simulink model "LAB9_PI"  (R2022b)
settings: Solver=VariableStepAuto  StartTime=0.0  StopTime=czas_systemu  RelTol=1e-3
values from neighbouring files (symbols this model uses):
  Cvp = cp*rop*Vp    (= 36000)    [LAB9.m]
  Cvw = cp*rop*Vw    (= 72000)    [LAB9.m]
  dqg = 0.1*q_g_N    (= 1000)    [LAB9.m]
  dTzew = 1    [LAB9.m]
  K_cp = ((a1*q_g_N)*(T_wew_N-Tp_N))/((Tp_N-T_zew_N)*(T_wew_N-T_zew_N+a1*(T_wew_N-Tp_N)))    (= 23.2558139535)    [LAB9.m]
  K_cw = (q_g_N)/(T_wew_N-T_zew_N+a1*(T_wew_N-Tp_N))    (= 232.558139535)    [LAB9.m]
  K_cwp = (a1*(q_g_N))/(T_wew_N-T_zew_N+a1*(T_wew_N-Tp_N))    (= 69.7674418605)    [LAB9.m]
  Kd = 0    [LAB9.m]
  Ki = Kp/(3.33*T_0_tp)    (= 9.00900900901)    [LAB9.m]
  Kp = (0.9*T_sp)/(ksTp*T_0_tp)    (= 3000)    [LAB9.m]
  L11 = [ksTwew]    [LAB9.m]
  L12 = [ksTp]    [LAB9.m]
  L21 = [kmdTwew]    [LAB9.m]
  L22 = [kmdTp]    [LAB9.m]
  M1 = [T,1]    [LAB9.m]
  M2 = [T_sp,1]    [LAB9.m]
  M3 = [T2,1]    [LAB9.m]
  M4 = [T3,1]    [LAB9.m]
  q_g_0 = K_cw*(T_wew_0-T_zew_0)+K_cwp*(T_wew_0-Tp_0)    (= 11666.6666667)    [LAB9.m]
  t0 = 1000    [LAB9.m]
  T_0_tp = 100    [LAB9.m]
  T_0_wew = 0    [LAB9.m]
  T_wew_0 = (K_cwp*Tp_0+K_cp*Tp_0-K_cp*T_zew_0)/K_cwp    (= 26.6666666667)    [LAB9.m]
  T_zew_0 = T_zew_N    (= -20)    [LAB9.m]
  To = t_2w-T2    (= 0)    [LAB9.m]
  To1 = t_2p-T3    (= 175)    [LAB9.m]
  Tp_0 = Tp_N+b    (= 15)    [LAB9.m]
  Tp_N = 10    [LAB9.m]
libraries: slpidlib x5
settings Model: Creator=maciejrudy  LastModifiedBy=Dawid
settings SolverCC: AlgebraicLoopSolver=TrustRegion
settings DataIOCC: ReturnWorkspaceOutputs=off
settings DebuggingCC: UnconnectedInputMsg=warning  UnconnectedOutputMsg=warning  UnconnectedLineMsg=warning  SFMachineParentedDataDiag=warning
settings ModelReferenceCC: EnableRefExpFcnMdlSchedulingChecks=on
settings RTWCC: DLArmComputeVersion=19.05

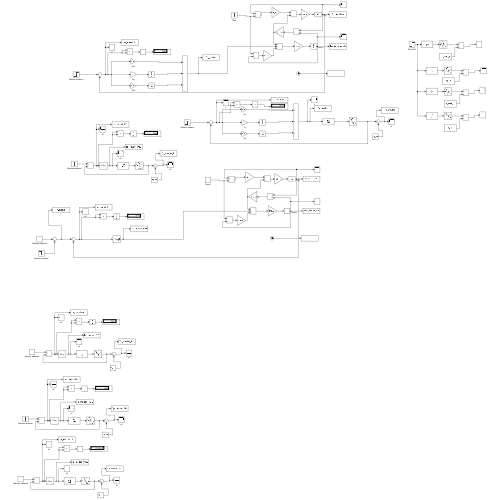
[thumbnail: Simulink's stored preview of the top-level diagram]
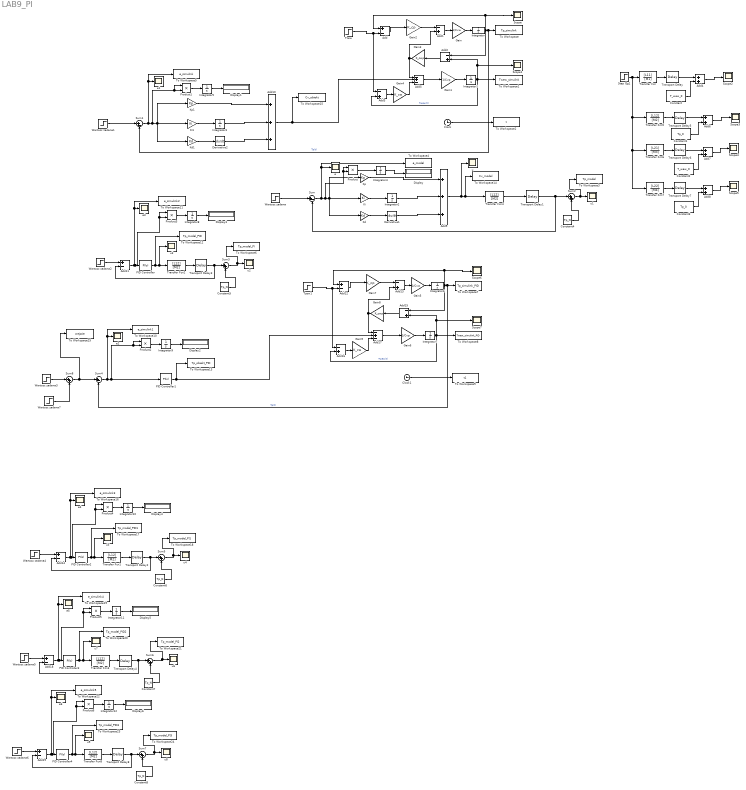
== system LAB9_PI ==
  Add{,11..12,14,18..19} (6 alike) : Sum  Inputs=+-
  Add{1..3,13,15..16} (6 alike) : Sum  Inputs=-+
  Add10 : Sum  Inputs=+++
  Add17 : Sum  Inputs=-+-
  Add{4,6..8} (4 alike) : Sum
  Add5 : Sum  Inputs=-+-
  Add9 : Sum  Inputs=+++
  Clock : Clock
  Clock1 : Clock
  Constant : Constant  Value=T_wew_0
  Constant1 : Constant  Value=Tp_0
  Constant2 : Constant  Value=T_wew_0
  Constant3 : Constant  Value=Tp_0
  Constant{4..8} (5 alike) : Constant  Value=Tp_N
  Derivative1 : Derivative
  Derivative2 : Derivative
  Display{,1..6} (7 alike) : Display
  Gain : Gain  Gain=1/Cvw
  Gain1 : Gain  Gain=1/Cvp
  Gain2 : Gain  Gain=K_cp
  Gain3 : Gain  Gain=K_cwp
  Gain4 : Gain  Gain=K_cw
  Gain5 : Gain  Gain=1/Cvw
  Gain6 : Gain  Gain=1/Cvp
  Gain7 : Gain  Gain=K_cp
  Gain8 : Gain  Gain=K_cwp
  Gain9 : Gain  Gain=K_cw
  Integrator : Integrator  InitialCondition=Tp_0
  Integrator1 : Integrator  InitialCondition=T_wew_0
  Integrator{2,4..5,8..12} (8 alike) : Integrator
  Integrator3 : Integrator  InitialCondition=q_g_0
  Integrator6 : Integrator  InitialCondition=Tp_0
  Integrator7 : Integrator  InitialCondition=T_wew_0
  Kd : Gain  Gain=Kd
  Kd1 : Gain  Gain=Kd
  Ki : Gain  Gain=Ki
  Ki1 : Gain  Gain=Ki
  Kp : Gain  Gain=Kp
  Kp1 : Gain  Gain=Kp
  PID Controller : slpidlib/PID Controller  Controller=PI  Form=Parallel  TimeDomain=Continuous-time  UseExternalTs=off  SampleTime=-1  IntegratorMethod=Forward Euler  FilterMethod=Forward Euler  ControllerParametersSource=internal  P=474.217741938703  I=1.00741516642566  UseKiTs=off  D=-0.04857589160968  N=3.78094165182863  UseFilter=on  TunerSelectOption=Transfer Function Based (PID Tuner App)  InitialConditionSource=internal  InitialConditionForIntegrator=0  InitialConditionForFilter=0  DifferentiatorICPrevScaledInput=0  ExternalReset=none  TrackingMode=off  Kt=1  LimitOutput=off  SatLimitsSource=internal  UpperSaturationLimit=inf  LowerSaturationLimit=-inf  LinearizeAsGain=on  AntiWindupMode=none  Kb=1  LimitIntegrator=off  UpperIntegratorSaturationLimit=inf  LowerIntegratorSaturationLimit=-inf  POutMin=[]  POutMax=[]  IOutMin=[]  IOutMax=[]  DOutMin=[]  DOutMax=[]  NOutMin=[]  NOutMax=[]  SumOutMin=[]  SumOutMax=[]  SaturationOutMin=[]  SaturationOutMax=[]  PParamMin=[]  PParamMax=[]  IParamMin=[]  IParamMax=[]  DParamMin=[]  DParamMax=[]  NParamMin=[]  NParamMax=[]  KbParamMin=[]  KbParamMax=[]  KtParamMin=[]  KtParamMax=[]  KbOutMin=[]  KbOutMax=[]  KtOutMin=[]  KtOutMax=[]  IntegratorOutMin=[]  IntegratorOutMax=[]  FilterOutMin=[]  FilterOutMax=[]  SumI1OutMin=[]  SumI1OutMax=[]  SumI2OutMin=[]  SumI2OutMax=[]  SumI3OutMin=[]  SumI3OutMax=[]  SumI4OutMin=[]  SumI4OutMax=[]  SumDOutMin=[]  SumDOutMax=[]  DifferentiatorOutMin=[]  DifferentiatorOutMax=[]  FilterDiffOutCoefMin=[]  FilterDiffOutCoefMax=[]  ReciprocalOutMin=[]  ReciprocalOutMax=[]  SumDenOutMin=[]  SumDenOutMax=[]  SumNumOutMin=[]  SumNumOutMax=[]  DivideOutMin=[]  DivideOutMax=[]  UdiffTsProdOutMin=[]  UdiffTsProdOutMax=[]  NTsProdOutMin=[]  NTsProdOutMax=[]  UintegralTsProdOutMin=[]  UintegralTsProdOutMax=[]  UngainTsProdOutMin=[]  UngainTsProdOutMax=[]  ClampingZeroOutDataTypeStr=Inherit: Inherit via back propagation  ClampingZeroOutMin=[]  ClampingZeroOutMax=[]  FilterDenConstantOutDataTypeStr=Inherit: Inherit via back propagation  FilterDenConstantOutMin=[]  FilterDenConstantOutMax=[]  PCopyOutDataTypeStr=Inherit: Inherit via back propagation  PCopyOutMin=[]  PCopyOutMax=[]  NCopyOutDataTypeStr=Inherit: Inherit via back propagation  NCopyOutMin=[]  NCopyOutMax=[]  IntegratorContinuousStateAttributes=''  IntegratorStateMustResolveToSignalObject=off  IntegratorRTWStateStorageClass=Auto  FilterContinuousStateAttributes=''  FilterStateMustResolveToSignalObject=off  FilterRTWStateStorageClass=Auto  ParallelPVariant=InternalParameters  IdealPVariant=Disabled  IVariant=InternalParameters  DVariant=Disabled  IntegratorVariant=Continuous  SatVariant=Disabled  AWVariant=Passthrough  PCopyVariant=Disabled  TRVariant=Disabled  FdbkBlocksVariant=Forward  IdealPFdbkVariant=Disabled  SatFdbkVariant=Disabled  DerivativeFilterVariant=Disabled  NVariant=Disabled  NCopyVariant=Disabled_SignalSpec  FilterICVariant=Disabled  IntegratorICVariant=InternalICs  ExternalResetVariant=Disabled  TRSumVariant=Passthrough  SumFdbkVariant=Disabled  SumVariant=Sum_PI  TsampFilterVariant=InternalTs  TsampNgainVariant=Passthrough  TsampIntegralVariant=Passthrough  ExternalSaturationOutDataTypeStr=Inherit: Same as second input
  PID Controller1 : slpidlib/PID Controller  Controller=PI  Form=Parallel  TimeDomain=Continuous-time  UseExternalTs=off  SampleTime=-1  IntegratorMethod=Forward Euler  FilterMethod=Forward Euler  ControllerParametersSource=internal  P=2025.02642427682  I=9.10127320670196  UseKiTs=off  D=-0.04857589160968  N=3.78094165182863  UseFilter=on  TunerSelectOption=Transfer Function Based (PID Tuner App)  InitialConditionSource=internal  InitialConditionForIntegrator=q_g_0  InitialConditionForFilter=0  DifferentiatorICPrevScaledInput=0  ExternalReset=none  TrackingMode=off  Kt=1  LimitOutput=on  SatLimitsSource=internal  UpperSaturationLimit=13000  LowerSaturationLimit=-inf  LinearizeAsGain=on  AntiWindupMode=back-calculation  Kb=2  LimitIntegrator=off  UpperIntegratorSaturationLimit=inf  LowerIntegratorSaturationLimit=-inf  POutMin=[]  POutMax=[]  IOutMin=[]  IOutMax=[]  DOutMin=[]  DOutMax=[]  NOutMin=[]  NOutMax=[]  SumOutMin=[]  SumOutMax=[]  SaturationOutMin=[]  SaturationOutMax=[]  PParamMin=[]  PParamMax=[]  IParamMin=[]  IParamMax=[]  DParamMin=[]  DParamMax=[]  NParamMin=[]  NParamMax=[]  KbParamMin=[]  KbParamMax=[]  KtParamMin=[]  KtParamMax=[]  KbOutMin=[]  KbOutMax=[]  KtOutMin=[]  KtOutMax=[]  IntegratorOutMin=[]  IntegratorOutMax=[]  FilterOutMin=[]  FilterOutMax=[]  SumI1OutMin=[]  SumI1OutMax=[]  SumI2OutMin=[]  SumI2OutMax=[]  SumI3OutMin=[]  SumI3OutMax=[]  SumI4OutMin=[]  SumI4OutMax=[]  SumDOutMin=[]  SumDOutMax=[]  DifferentiatorOutMin=[]  DifferentiatorOutMax=[]  FilterDiffOutCoefMin=[]  FilterDiffOutCoefMax=[]  ReciprocalOutMin=[]  ReciprocalOutMax=[]  SumDenOutMin=[]  SumDenOutMax=[]  SumNumOutMin=[]  SumNumOutMax=[]  DivideOutMin=[]  DivideOutMax=[]  UdiffTsProdOutMin=[]  UdiffTsProdOutMax=[]  NTsProdOutMin=[]  NTsProdOutMax=[]  UintegralTsProdOutMin=[]  UintegralTsProdOutMax=[]  UngainTsProdOutMin=[]  UngainTsProdOutMax=[]  ClampingZeroOutDataTypeStr=Inherit: Inherit via back propagation  ClampingZeroOutMin=[]  ClampingZeroOutMax=[]  FilterDenConstantOutDataTypeStr=Inherit: Inherit via back propagation  FilterDenConstantOutMin=[]  FilterDenConstantOutMax=[]  PCopyOutDataTypeStr=Inherit: Inherit via back propagation  PCopyOutMin=[]  PCopyOutMax=[]  NCopyOutDataTypeStr=Inherit: Inherit via back propagation  NCopyOutMin=[]  NCopyOutMax=[]  IntegratorContinuousStateAttributes=''  IntegratorStateMustResolveToSignalObject=off  IntegratorRTWStateStorageClass=Auto  FilterContinuousStateAttributes=''  FilterStateMustResolveToSignalObject=off  FilterRTWStateStorageClass=Auto  ParallelPVariant=InternalParameters  IdealPVariant=Disabled  IVariant=InternalParameters  DVariant=Disabled  IntegratorVariant=Continuous  SatVariant=Enabled  AWVariant=BackCalculation  PCopyVariant=Disabled  TRVariant=Disabled  FdbkBlocksVariant=Forward  IdealPFdbkVariant=Disabled  SatFdbkVariant=Disabled  DerivativeFilterVariant=Disabled  NVariant=Disabled  NCopyVariant=Disabled_SignalSpec  FilterICVariant=Disabled  IntegratorICVariant=InternalICs  ExternalResetVariant=Disabled  TRSumVariant=Passthrough  SumFdbkVariant=Disabled  SumVariant=Sum_PI  TsampFilterVariant=InternalTs  TsampNgainVariant=Passthrough  TsampIntegralVariant=Passthrough  ExternalSaturationOutDataTypeStr=Inherit: Same as second input
  PID Controller2 : slpidlib/PID Controller  Controller=PI  Form=Parallel  TimeDomain=Continuous-time  UseExternalTs=off  SampleTime=-1  IntegratorMethod=Forward Euler  FilterMethod=Forward Euler  ControllerParametersSource=internal  P=2098.51287739334  I=0.228001720884021  UseKiTs=off  D=-0.04857589160968  N=3.78094165182863  UseFilter=on  TunerSelectOption=Transfer Function Based (PID Tuner App)  InitialConditionSource=internal  InitialConditionForIntegrator=0  InitialConditionForFilter=0  DifferentiatorICPrevScaledInput=0  ExternalReset=none  TrackingMode=off  Kt=1  LimitOutput=off  SatLimitsSource=internal  UpperSaturationLimit=inf  LowerSaturationLimit=-inf  LinearizeAsGain=on  AntiWindupMode=none  Kb=1  LimitIntegrator=off  UpperIntegratorSaturationLimit=inf  LowerIntegratorSaturationLimit=-inf  POutMin=[]  POutMax=[]  IOutMin=[]  IOutMax=[]  DOutMin=[]  DOutMax=[]  NOutMin=[]  NOutMax=[]  SumOutMin=[]  SumOutMax=[]  SaturationOutMin=[]  SaturationOutMax=[]  PParamMin=[]  PParamMax=[]  IParamMin=[]  IParamMax=[]  DParamMin=[]  DParamMax=[]  NParamMin=[]  NParamMax=[]  KbParamMin=[]  KbParamMax=[]  KtParamMin=[]  KtParamMax=[]  KbOutMin=[]  KbOutMax=[]  KtOutMin=[]  KtOutMax=[]  IntegratorOutMin=[]  IntegratorOutMax=[]  FilterOutMin=[]  FilterOutMax=[]  SumI1OutMin=[]  SumI1OutMax=[]  SumI2OutMin=[]  SumI2OutMax=[]  SumI3OutMin=[]  SumI3OutMax=[]  SumI4OutMin=[]  SumI4OutMax=[]  SumDOutMin=[]  SumDOutMax=[]  DifferentiatorOutMin=[]  DifferentiatorOutMax=[]  FilterDiffOutCoefMin=[]  FilterDiffOutCoefMax=[]  ReciprocalOutMin=[]  ReciprocalOutMax=[]  SumDenOutMin=[]  SumDenOutMax=[]  SumNumOutMin=[]  SumNumOutMax=[]  DivideOutMin=[]  DivideOutMax=[]  UdiffTsProdOutMin=[]  UdiffTsProdOutMax=[]  NTsProdOutMin=[]  NTsProdOutMax=[]  UintegralTsProdOutMin=[]  UintegralTsProdOutMax=[]  UngainTsProdOutMin=[]  UngainTsProdOutMax=[]  ClampingZeroOutDataTypeStr=Inherit: Inherit via back propagation  ClampingZeroOutMin=[]  ClampingZeroOutMax=[]  FilterDenConstantOutDataTypeStr=Inherit: Inherit via back propagation  FilterDenConstantOutMin=[]  FilterDenConstantOutMax=[]  PCopyOutDataTypeStr=Inherit: Inherit via back propagation  PCopyOutMin=[]  PCopyOutMax=[]  NCopyOutDataTypeStr=Inherit: Inherit via back propagation  NCopyOutMin=[]  NCopyOutMax=[]  IntegratorContinuousStateAttributes=''  IntegratorStateMustResolveToSignalObject=off  IntegratorRTWStateStorageClass=Auto  FilterContinuousStateAttributes=''  FilterStateMustResolveToSignalObject=off  FilterRTWStateStorageClass=Auto  ParallelPVariant=InternalParameters  IdealPVariant=Disabled  IVariant=InternalParameters  DVariant=Disabled  IntegratorVariant=Continuous  SatVariant=Disabled  AWVariant=Passthrough  PCopyVariant=Disabled  TRVariant=Disabled  FdbkBlocksVariant=Forward  IdealPFdbkVariant=Disabled  SatFdbkVariant=Disabled  DerivativeFilterVariant=Disabled  NVariant=Disabled  NCopyVariant=Disabled_SignalSpec  FilterICVariant=Disabled  IntegratorICVariant=InternalICs  ExternalResetVariant=Disabled  TRSumVariant=Passthrough  SumFdbkVariant=Disabled  SumVariant=Sum_PI  TsampFilterVariant=InternalTs  TsampNgainVariant=Passthrough  TsampIntegralVariant=Passthrough  ExternalSaturationOutDataTypeStr=Inherit: Same as second input
  PID Controller3 : slpidlib/PID Controller  Controller=PI  Form=Parallel  TimeDomain=Continuous-time  UseExternalTs=off  SampleTime=-1  IntegratorMethod=Forward Euler  FilterMethod=Forward Euler  ControllerParametersSource=internal  P=474.217741938703  I=1.00741516642566  UseKiTs=off  D=-0.04857589160968  N=3.78094165182863  UseFilter=on  TunerSelectOption=Transfer Function Based (PID Tuner App)  InitialConditionSource=internal  InitialConditionForIntegrator=0  InitialConditionForFilter=0  DifferentiatorICPrevScaledInput=0  ExternalReset=none  TrackingMode=off  Kt=1  LimitOutput=off  SatLimitsSource=internal  UpperSaturationLimit=inf  LowerSaturationLimit=-inf  LinearizeAsGain=on  AntiWindupMode=none  Kb=1  LimitIntegrator=off  UpperIntegratorSaturationLimit=inf  LowerIntegratorSaturationLimit=-inf  POutMin=[]  POutMax=[]  IOutMin=[]  IOutMax=[]  DOutMin=[]  DOutMax=[]  NOutMin=[]  NOutMax=[]  SumOutMin=[]  SumOutMax=[]  SaturationOutMin=[]  SaturationOutMax=[]  PParamMin=[]  PParamMax=[]  IParamMin=[]  IParamMax=[]  DParamMin=[]  DParamMax=[]  NParamMin=[]  NParamMax=[]  KbParamMin=[]  KbParamMax=[]  KtParamMin=[]  KtParamMax=[]  KbOutMin=[]  KbOutMax=[]  KtOutMin=[]  KtOutMax=[]  IntegratorOutMin=[]  IntegratorOutMax=[]  FilterOutMin=[]  FilterOutMax=[]  SumI1OutMin=[]  SumI1OutMax=[]  SumI2OutMin=[]  SumI2OutMax=[]  SumI3OutMin=[]  SumI3OutMax=[]  SumI4OutMin=[]  SumI4OutMax=[]  SumDOutMin=[]  SumDOutMax=[]  DifferentiatorOutMin=[]  DifferentiatorOutMax=[]  FilterDiffOutCoefMin=[]  FilterDiffOutCoefMax=[]  ReciprocalOutMin=[]  ReciprocalOutMax=[]  SumDenOutMin=[]  SumDenOutMax=[]  SumNumOutMin=[]  SumNumOutMax=[]  DivideOutMin=[]  DivideOutMax=[]  UdiffTsProdOutMin=[]  UdiffTsProdOutMax=[]  NTsProdOutMin=[]  NTsProdOutMax=[]  UintegralTsProdOutMin=[]  UintegralTsProdOutMax=[]  UngainTsProdOutMin=[]  UngainTsProdOutMax=[]  ClampingZeroOutDataTypeStr=Inherit: Inherit via back propagation  ClampingZeroOutMin=[]  ClampingZeroOutMax=[]  FilterDenConstantOutDataTypeStr=Inherit: Inherit via back propagation  FilterDenConstantOutMin=[]  FilterDenConstantOutMax=[]  PCopyOutDataTypeStr=Inherit: Inherit via back propagation  PCopyOutMin=[]  PCopyOutMax=[]  NCopyOutDataTypeStr=Inherit: Inherit via back propagation  NCopyOutMin=[]  NCopyOutMax=[]  IntegratorContinuousStateAttributes=''  IntegratorStateMustResolveToSignalObject=off  IntegratorRTWStateStorageClass=Auto  FilterContinuousStateAttributes=''  FilterStateMustResolveToSignalObject=off  FilterRTWStateStorageClass=Auto  ParallelPVariant=InternalParameters  IdealPVariant=Disabled  IVariant=InternalParameters  DVariant=Disabled  IntegratorVariant=Continuous  SatVariant=Disabled  AWVariant=Passthrough  PCopyVariant=Disabled  TRVariant=Disabled  FdbkBlocksVariant=Forward  IdealPFdbkVariant=Disabled  SatFdbkVariant=Disabled  DerivativeFilterVariant=Disabled  NVariant=Disabled  NCopyVariant=Disabled_SignalSpec  FilterICVariant=Disabled  IntegratorICVariant=InternalICs  ExternalResetVariant=Disabled  TRSumVariant=Passthrough  SumFdbkVariant=Disabled  SumVariant=Sum_PI  TsampFilterVariant=InternalTs  TsampNgainVariant=Passthrough  TsampIntegralVariant=Passthrough  ExternalSaturationOutDataTypeStr=Inherit: Same as second input
  PID Controller4 : slpidlib/PID Controller  Controller=PI  Form=Parallel  TimeDomain=Continuous-time  UseExternalTs=off  SampleTime=-1  IntegratorMethod=Forward Euler  FilterMethod=Forward Euler  ControllerParametersSource=internal  P=4975.52155708983  I=1.2967764011039  UseKiTs=off  D=-0.04857589160968  N=3.78094165182863  UseFilter=on  TunerSelectOption=Transfer Function Based (PID Tuner App)  InitialConditionSource=internal  InitialConditionForIntegrator=0  InitialConditionForFilter=0  DifferentiatorICPrevScaledInput=0  ExternalReset=none  TrackingMode=off  Kt=1  LimitOutput=off  SatLimitsSource=internal  UpperSaturationLimit=inf  LowerSaturationLimit=-inf  LinearizeAsGain=on  AntiWindupMode=none  Kb=1  LimitIntegrator=off  UpperIntegratorSaturationLimit=inf  LowerIntegratorSaturationLimit=-inf  POutMin=[]  POutMax=[]  IOutMin=[]  IOutMax=[]  DOutMin=[]  DOutMax=[]  NOutMin=[]  NOutMax=[]  SumOutMin=[]  SumOutMax=[]  SaturationOutMin=[]  SaturationOutMax=[]  PParamMin=[]  PParamMax=[]  IParamMin=[]  IParamMax=[]  DParamMin=[]  DParamMax=[]  NParamMin=[]  NParamMax=[]  KbParamMin=[]  KbParamMax=[]  KtParamMin=[]  KtParamMax=[]  KbOutMin=[]  KbOutMax=[]  KtOutMin=[]  KtOutMax=[]  IntegratorOutMin=[]  IntegratorOutMax=[]  FilterOutMin=[]  FilterOutMax=[]  SumI1OutMin=[]  SumI1OutMax=[]  SumI2OutMin=[]  SumI2OutMax=[]  SumI3OutMin=[]  SumI3OutMax=[]  SumI4OutMin=[]  SumI4OutMax=[]  SumDOutMin=[]  SumDOutMax=[]  DifferentiatorOutMin=[]  DifferentiatorOutMax=[]  FilterDiffOutCoefMin=[]  FilterDiffOutCoefMax=[]  ReciprocalOutMin=[]  ReciprocalOutMax=[]  SumDenOutMin=[]  SumDenOutMax=[]  SumNumOutMin=[]  SumNumOutMax=[]  DivideOutMin=[]  DivideOutMax=[]  UdiffTsProdOutMin=[]  UdiffTsProdOutMax=[]  NTsProdOutMin=[]  NTsProdOutMax=[]  UintegralTsProdOutMin=[]  UintegralTsProdOutMax=[]  UngainTsProdOutMin=[]  UngainTsProdOutMax=[]  ClampingZeroOutDataTypeStr=Inherit: Inherit via back propagation  ClampingZeroOutMin=[]  ClampingZeroOutMax=[]  FilterDenConstantOutDataTypeStr=Inherit: Inherit via back propagation  FilterDenConstantOutMin=[]  FilterDenConstantOutMax=[]  PCopyOutDataTypeStr=Inherit: Inherit via back propagation  PCopyOutMin=[]  PCopyOutMax=[]  NCopyOutDataTypeStr=Inherit: Inherit via back propagation  NCopyOutMin=[]  NCopyOutMax=[]  IntegratorContinuousStateAttributes=''  IntegratorStateMustResolveToSignalObject=off  IntegratorRTWStateStorageClass=Auto  FilterContinuousStateAttributes=''  FilterStateMustResolveToSignalObject=off  FilterRTWStateStorageClass=Auto  ParallelPVariant=InternalParameters  IdealPVariant=Disabled  IVariant=InternalParameters  DVariant=Disabled  IntegratorVariant=Continuous  SatVariant=Disabled  AWVariant=Passthrough  PCopyVariant=Disabled  TRVariant=Disabled  FdbkBlocksVariant=Forward  IdealPFdbkVariant=Disabled  SatFdbkVariant=Disabled  DerivativeFilterVariant=Disabled  NVariant=Disabled  NCopyVariant=Disabled_SignalSpec  FilterICVariant=Disabled  IntegratorICVariant=InternalICs  ExternalResetVariant=Disabled  TRSumVariant=Passthrough  SumFdbkVariant=Disabled  SumVariant=Sum_PI  TsampFilterVariant=InternalTs  TsampNgainVariant=Passthrough  TsampIntegralVariant=Passthrough  ExternalSaturationOutDataTypeStr=Inherit: Same as second input
  Product{,1..6} (7 alike) : Product
  Scope{,1..7} (8 alike) : Scope
  Step Qg1 : Step  Time=t0  After=dqg  SampleTime=0
  Sum : Sum  Inputs=|+-
  Sum1 : Sum  Inputs=|+-
  Sum{2..3,5..8} (6 alike) : Sum  Inputs=|++
  Sum4 : Sum  Inputs=|+-
  To Workspace : ToWorkspace  VariableName=Tp_simulink  SampleTime=-1
  To Workspace1 : ToWorkspace  VariableName=Twew_simulink  SampleTime=-1
  To Workspace10 : ToWorkspace  VariableName=e_simulink1  SampleTime=-1
  To Workspace11 : ToWorkspace  VariableName=e_simulink2  SampleTime=-1
  To Workspace12 : ToWorkspace  VariableName=Tp_model_PID  SampleTime=-1
  To Workspace13 : ToWorkspace  VariableName=Tp_obiekt_PID  SampleTime=-1
  To Workspace14 : ToWorkspace  VariableName=Cv_model  SampleTime=-1
  To Workspace15 : ToWorkspace  VariableName=Cv_obiekt  SampleTime=-1
  To Workspace16 : ToWorkspace  VariableName=e_simulink3  SampleTime=-1
  To Workspace17 : ToWorkspace  VariableName=Tp_model_PID1  SampleTime=-1
  To Workspace18 : ToWorkspace  VariableName=Tp_model_PI1  SampleTime=-1
  To Workspace19 : ToWorkspace  VariableName=e_simulink4  SampleTime=-1
  To Workspace2 : ToWorkspace  VariableName=t  SaveFormat=Timeseries  SampleTime=-1
  To Workspace20 : ToWorkspace  VariableName=Tp_model_PID2  SampleTime=-1
  To Workspace21 : ToWorkspace  VariableName=Tp_model_PI2  SampleTime=-1
  To Workspace22 : ToWorkspace  VariableName=e_simulink5  SampleTime=-1
  To Workspace23 : ToWorkspace  VariableName=Tp_model_PID3  SampleTime=-1
  To Workspace24 : ToWorkspace  VariableName=Tp_model_PI3  SampleTime=-1
  To Workspace25 : ToWorkspace  VariableName=wejscie  SampleTime=-1
  To Workspace3 : ToWorkspace  VariableName=Tp_model  SampleTime=-1
  To Workspace4 : ToWorkspace  VariableName=e_model  SampleTime=-1
  To Workspace5 : ToWorkspace  VariableName=e_simulink  SampleTime=-1
  To Workspace6 : ToWorkspace  VariableName=Tp_model_PI  SampleTime=-1
  To Workspace7 : ToWorkspace  VariableName=Tp_simulink_PID  SampleTime=-1
  To Workspace8 : ToWorkspace  VariableName=Twew_simulink_PID  SampleTime=-1
  To Workspace9 : ToWorkspace  VariableName=t1  SaveFormat=Timeseries  SampleTime=-1
  Transfer Fcn : TransferFcn  Numerator=[L11]  Denominator=[M1]
  Transfer Fcn{1..5,8} (6 alike) : TransferFcn  Numerator=[L12]  Denominator=[M2]
  Transfer Fcn6 : TransferFcn  Numerator=[L21]  Denominator=[M3]
  Transfer Fcn7 : TransferFcn  Numerator=[L22]  Denominator=[M4]
  Transport Delay : TransportDelay  DelayTime=T_0_wew
  Transport Delay{1..5,8} (6 alike) : TransportDelay  DelayTime=T_0_tp
  Transport Delay6 : TransportDelay  DelayTime=To
  Transport Delay7 : TransportDelay  DelayTime=To1
  Tzew : Step  Time=t0  Before=T_zew_0  After=T_zew_0+dTzew  SampleTime=0
  Tzew1 : Step  Time=t0  Before=T_zew_0  After=T_zew_0+dTzew  SampleTime=0
  Wartosc zadana{,2,4..6} (5 alike) : Step  Time=t0  After=2  SampleTime=0
  Wartosc zadana1 : Step  Time=t0  Before=Tp_0  After=Tp_0+2  SampleTime=0
  Wartosc zadana3 : Step  Time=t0+2000  Before=Tp_0  After=Tp_0+dTzew  SampleTime=0
  Wartosc zadana7 : Step  Time=t0+8000  After=-dTzew  SampleTime=0
  e{,1..6} (7 alike) : Scope
  u{,1..9} (10 alike) : Scope
  wires:
  Wartosc zadana/1 -> Sum/1
  Transfer Fcn4/1 -> Transport Delay1/1
  Transport Delay6/1 -> Add7/1
  Add9/1 -> u/1, To Workspace14/1, Transfer Fcn4/1
  Gain3/1 -> Add5/1, Add1/2
  Add4/1 -> Scope2/1
  Gain/1 -> Integrator/1
  Transport Delay7/1 -> Add8/1
  Add2/1 -> Gain3/1
  Constant1/1 -> Add6/2
  Add5/1 -> Gain1/1
  Constant/1 -> Add4/2
  Gain4/1 -> Add5/3
  Gain1/1 -> Integrator1/1
  Integrator/1 -> Add2/1, To Workspace/1, Sum1/2, Scope/1, Add/1  "Tp(t)"
  Transfer Fcn5/1 -> Transport Delay5/1
  Add8/1 -> Scope5/1
  Add1/1 -> Gain/1
  Transport Delay/1 -> Add4/1
  Step Qg1/1 -> Transfer Fcn5/1, Transfer Fcn7/1, Transfer Fcn6/1, Transfer Fcn/1
  Transfer Fcn7/1 -> Transport Delay7/1
  Clock/1 -> To Workspace2/1
  Add/1 -> Gain2/1
  Integrator1/1 -> Add3/2, To Workspace1/1, Add2/2, Scope1/1  "Twew(t)"
  Add3/1 -> Gain4/1
  Transport Delay5/1 -> Add6/1
  Constant2/1 -> Add7/2
  Transfer Fcn/1 -> Transport Delay/1
  Add7/1 -> Scope4/1
  Tzew/1 -> Add3/1, Add/2
  Constant3/1 -> Add8/2
  Ki/1 -> Integrator2/1
  Add6/1 -> Scope3/1
  Gain2/1 -> Add1/1
  Integrator2/1 -> Add9/2
  Transfer Fcn6/1 -> Transport Delay6/1
  Sum/1 -> Ki/1, Kp/1, Kd/1, Product/1, Product/2, To Workspace4/1, e/1
  Kp/1 -> Add9/1
  Kd/1 -> Derivative1/1
  Derivative1/1 -> Add9/3
  Transport Delay1/1 -> Sum/2, Sum2/1
  Sum1/1 -> To Workspace5/1, e1/1, Ki1/1, Kp1/1, Kd1/1, Product1/1, Product1/2
  Integrator3/1 -> Add10/2
  Kd1/1 -> Derivative2/1
  Derivative2/1 -> Add10/3
  Kp1/1 -> Add10/1
  Ki1/1 -> Integrator3/1
  Wartosc zadana1/1 -> Sum1/1
  Add10/1 -> To Workspace15/1, Add5/2
  Product/1 -> Integrator4/1
  Integrator4/1 -> Display/1
  Product1/1 -> Integrator5/1
  Integrator5/1 -> Display1/1
  Sum2/1 -> To Workspace3/1, u1/1
  Constant4/1 -> Sum2/2
  Wartosc zadana2/1 -> Add11/1
  PID Controller/1 -> To Workspace12/1, u3/1, Transfer Fcn2/1
  Transfer Fcn2/1 -> Transport Delay3/1
  Sum3/1 -> To Workspace6/1, u2/1
  Constant5/1 -> Sum3/2
  Transport Delay3/1 -> Add11/2, Sum3/1
  Gain8/1 -> Add17/1, Add13/2
  Integrator9/1 -> Display2/1
  Gain6/1 -> Integrator7/1
  Add15/1 -> Gain8/1
  Product2/1 -> Integrator9/1
  Tzew1/1 -> Add16/1, Add12/2
  Add12/1 -> Gain7/1
  Gain5/1 -> Integrator6/1
  Gain7/1 -> Add13/1
  Gain9/1 -> Add17/3
  Integrator7/1 -> Add16/2, To Workspace8/1, Add15/2, Scope7/1  "Twew(t)"
  Clock1/1 -> To Workspace9/1
  Sum4/1 -> To Workspace10/1, e2/1, PID Controller1/1, Product2/1, Product2/2
  Add13/1 -> Gain5/1
  Add16/1 -> Gain9/1
  Add17/1 -> Gain6/1
  Integrator6/1 -> Add15/1, To Workspace7/1, Sum4/2, Scope6/1, Add12/1  "Tp(t)"
  PID Controller1/1 -> To Workspace13/1, Add17/2
  Add11/1 -> To Workspace11/1, e3/1, Product3/1, Product3/2, PID Controller/1
  Integrator8/1 -> Display3/1
  Product3/1 -> Integrator8/1
  Integrator10/1 -> Display4/1
  Product4/1 -> Integrator10/1
  Transport Delay2/1 -> Add14/2, Sum5/1
  Transfer Fcn1/1 -> Transport Delay2/1
  Add14/1 -> To Workspace16/1, e4/1, Product4/1, Product4/2, PID Controller2/1
  Wartosc zadana4/1 -> Add14/1
  PID Controller2/1 -> To Workspace17/1, u5/1, Transfer Fcn1/1
  Constant6/1 -> Sum5/2
  Sum5/1 -> To Workspace18/1, u4/1
  Integrator11/1 -> Display5/1
  Product5/1 -> Integrator11/1
  Transport Delay4/1 -> Add18/2, Sum6/1
  Transfer Fcn3/1 -> Transport Delay4/1
  Add18/1 -> To Workspace19/1, e5/1, Product5/1, Product5/2, PID Controller3/1
  Wartosc zadana5/1 -> Add18/1
  PID Controller3/1 -> To Workspace20/1, u7/1, Transfer Fcn3/1
  Constant7/1 -> Sum6/2
  Sum6/1 -> To Workspace21/1, u6/1
  Integrator12/1 -> Display6/1
  Product6/1 -> Integrator12/1
  Transport Delay8/1 -> Add19/2, Sum7/1
  Transfer Fcn8/1 -> Transport Delay8/1
  Add19/1 -> To Workspace22/1, e6/1, Product6/1, Product6/2, PID Controller4/1
  Wartosc zadana6/1 -> Add19/1
  PID Controller4/1 -> To Workspace23/1, u9/1, Transfer Fcn8/1
  Constant8/1 -> Sum7/2
  Sum7/1 -> To Workspace24/1, u8/1
  Wartosc zadana3/1 -> Sum8/1
  Wartosc zadana7/1 -> Sum8/2
  Sum8/1 -> To Workspace25/1, Sum4/1
